simulink model "harmonic_drive_paper"  (R2022b)
settings: Solver=VariableStepAuto  StartTime=0.0  StopTime=10.0  RelTol=1e-3
settings Model: Creator=saayu  LastModifiedBy=saayu

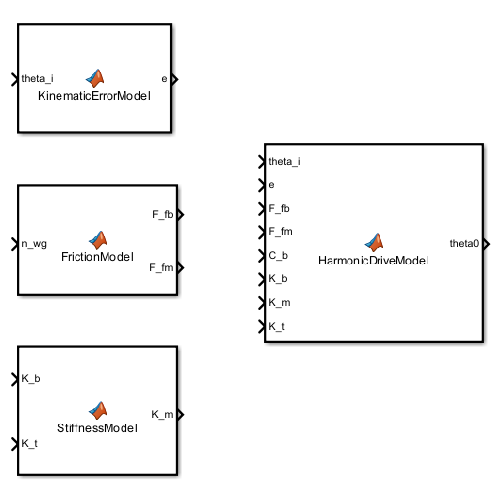
[thumbnail: Simulink's stored preview of the top-level diagram]
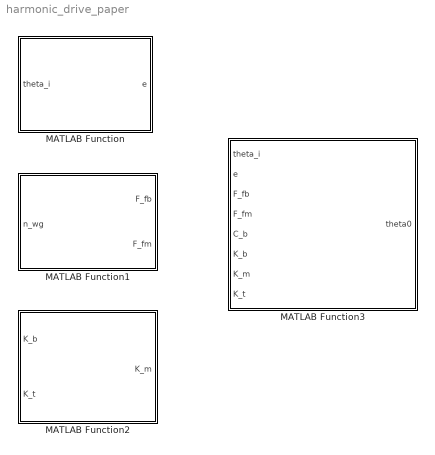
== system harmonic_drive_paper ==
  MATLAB Function : MATLAB Function  TreatAsAtomicUnit=on
  MATLAB Function1 : MATLAB Function  TreatAsAtomicUnit=on
  MATLAB Function2 : MATLAB Function  TreatAsAtomicUnit=on
  MATLAB Function3 : MATLAB Function  TreatAsAtomicUnit=on

== matlab function harmonic_drive_paper/MATLAB Function1 ==
  data: n_wg input; F_fb output; F_fm output
function [F_fb, F_fm] = FrictionModel(n_wg)

r_g = 0.03525;
alpha_t = 20;
f0 = 1.45;
v0 = 8e-5;
d_m = 0.058;
F_c = 6.43;
c = 6.72e-4;

c_si = c * 60 / (2 * pi);
alpha_t_rad = alpha_t * pi / 180;


F_fb = 1e-7 * f0 * (v0 * n_wg)^(2/3) * d_m^3 * sign(n_wg) / r_g;

F_fm = (F_c + c_si * n_wg) * sign(n_wg);

T_f = F_fb * r_g + F_fm * r_g * sin(alpha_t_rad);

== matlab function harmonic_drive_paper/MATLAB Function ==
  data: theta_i input; e output
function e = KinematicErrorModel(theta_i)

a0 = 0.4615e-3;
a1 = 0.2057e-3;
a2 = 0.011e-3;
b1 = 4.5e-3;
b2 = -1e-3;
w1 = 2;
w2 = 4;
r_g = 0.03525;
alpha_t = 20;

theta_i_rad = theta_i * pi / 180;
alpha_t_rad = alpha_t * pi / 180;


theta_ke_rec = (a0 / 2 + a1 * cos(w1 * theta_i_rad) + a2 * cos(w2 * theta_i_rad) + b1 * sin(w1 * theta_i_rad) + b2 * sin(w2 * theta_i_rad)) * pi / 180;

e = theta_ke_rec * r_g / tan(alpha_t_rad);

== matlab function harmonic_drive_paper/MATLAB Function2 ==
  data: K_b input; K_m output; K_t input
function K_m = StiffnessModel(K_b, K_t)

r_g = 0.03525;
alpha_t = 20;
g1 = 1.756e-5;
g2 = 1.95e-5;

alpha_t_rad = alpha_t * pi / 180;


T0 = K_t * (y_1 - y_2) / r_g;

delta_theta0 = g1 * T0^(1/3) + g2 * T0;

f_t = 1 / K_t;

f_b = 1 / (K_b * r_g^2 * cot(alpha_t_rad)^2);

f_m = g1 / (3 * T0^(2/3)) + g2 - f_t - f_b;

K_m = 1 / (f_m * r_g^2 * cos(alpha_t_rad)^2);

f_HD = f_m + f_t + f_b;

== matlab function harmonic_drive_paper/MATLAB Function3 ==
  data: theta_i input; e input; theta0 output; F_fb input; F_fm input; C_b input; K_b input; K_m input; K_t input
function theta0 = HarmonicDriveModel(theta_i, e, F_fb, F_fm, C_b, K_b, K_m, K_t)

r_g = 0.03525;
N = 50;
alpha_t = 20;
J_g = 2.57e-7;
J_o = 2.55e-3;
